simulink model "adaptive_beamforming"  (R2026a)
settings: Solver=VariableStepAuto  StopTime=60
libraries: dspstat3 x2, commchan3 x1, commfilt2 x1, commrandsrc3 x1, commdigbbndam3 x1
settings Model: PacingRate=4  Creator=Krrrrish  LastModifiedBy=swaja

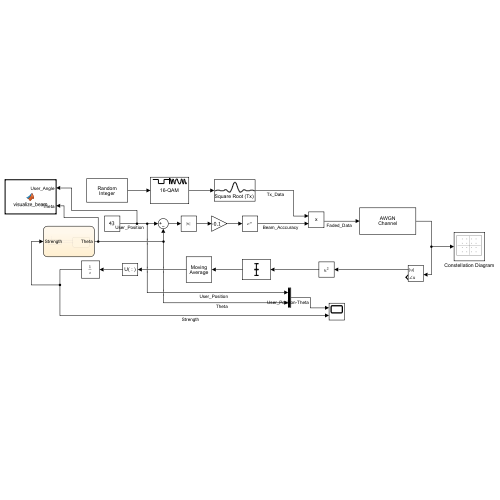
[thumbnail: Simulink's stored preview of the top-level diagram]
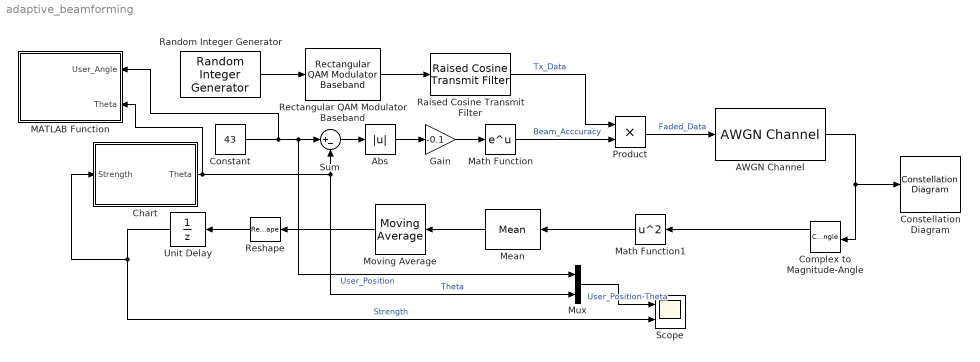
== system adaptive_beamforming ==
  AWGN Channel : commchan3/AWGN Channel  LegacyMode=off  NoiseMethod="Signal to noise ratio  (SNR)"  noiseMode="Signal to noise ratio  (SNR)"  EbNo=10  EsNo=10  SNR=10  BitsPerSymbol=1  SignalPower=1  SpecifySymbolPeriod=off  SamplesPerSymbol=1  SymbolPeriod=1  VarianceSource=Parameter  Variance=1  RandomStream=Global stream  Seed=67  SimulateUsing=Code generation
  Abs : Abs  SaturateOnIntegerOverflow=off
  Chart : Stateflow chart  TreatAsAtomicUnit=on
  Complex to Magnitude-Angle : ComplexToMagnitudeAngle
  Constant : Constant  Value=43
  Constellation Diagram : ConstellationDiagram  WindowPosition=[1071.000000,156.000000,600.000000,600.000000,]  ScopeFrameLocation=window  DefaultConfigurationName=comm.scopes.ConstellationDiagramBlockCfg
  Gain : Gain  Gain=-0.1
  MATLAB Function : MATLAB Function  TreatAsAtomicUnit=on
  Math Function : Math
  Math Function1 : Math  Operator=square
  Mean : dspstat3/Mean  run=off  InputProcessing=Columns as channels (frame based)  reset_popup=None  directionMode=Each column  dimension=1  roiEnable=off  roiType=Rectangles  roiPortion=Entire ROI  roiOutput=Individual statistics for each ROI  roiFlag=off  roundingMode=Floor  overflowMode=off  outputMin=[]  outputMax=[]
  Moving Average : dspstat3/Moving Average  Method=Sliding window  ForgettingFactorPort=off  SpecifyWindowLength=on  WindowLengthSource=Property  MaxWindowLength=20  WindowLength=4  OverlapLength=3  AllowArbitraryInputLength=off  ForgettingFactor=0.9  SimulateUsing=Interpreted execution
  Mux : Mux  Inputs=2
  Product : Product
  Raised Cosine Transmit Filter : commfilt2/Raised Cosine Transmit Filter  filtType=Square root  R=0.2  filtSpan=10  N=8  filterGain=1  InputProcessing=Columns as channels (frame based)  RateOptions=Enforce single-rate processing  framing=Mute  checkCoeff=off  variableName=rcTxFilt  checkGain=Normalized  sampMode=Mute  saveAsFlag=0  currentFiltSpan=10  D=(10)/2  launchFVT=on  roundingMode=Floor  overflowMode=off  coeffDataTypeStr=Inherit: Same word length as input  coeffMin=[]  coeffMax=[]  coeffLastDataTypeStr=Inherit: Same word length as input  outputDataTypeStr=Inherit: Same as accumulator  outputMin=[]  outputMax=[]  outputLastDataTypeStr=Inherit: Same as accumulator
  Random Integer Generator : commrandsrc3/Random Integer Generator  SetSize=8  SeedSource=Auto  Seed=0  SampleTime=1  SamplesPerFrame=1  OutputDataType=double  SimulateUsing=Interpreted execution
  Rectangular QAM Modulator Baseband : commdigbbndam3/Rectangular QAM Modulator Baseband  M=16  InType=Integer  Enc=Gray  Mapping=[0:15]  PowType=Min. distance between symbols  MinDist=2  AvgPow=1  PeakPow=1  Ph=0  outDtype=double  outWordLen=16  outUDDataType=sfix(16)  outFracLenMode=Best precision  outFracLen=15  outDataTypeStr=double  outLastDataTypeStr=double
  Reshape : Reshape
  Scope : Scope  NumInputPorts=2
      settings: ActiveDisplayYMinimum=-130.96926801320939  ActiveDisplayYMaximum=619.509013291859
  Sum : Sum  Inputs=|+-
  Unit Delay : UnitDelay  SampleTime=0.01
  wires:
  Random Integer Generator/1 -> Rectangular QAM Modulator Baseband/1
  Rectangular QAM Modulator Baseband/1 -> Raised Cosine Transmit Filter/1
  Raised Cosine Transmit Filter/1 -> Product/1  "Tx_Data"
  Chart/1(Theta) -> MATLAB Function/2(Theta), Mux/2, Sum/2  "Theta"
  Constant/1 -> MATLAB Function/1(User_Angle), Mux/1, Sum/1  "User_Position"
  Sum/1 -> Abs/1
  Abs/1 -> Gain/1
  Gain/1 -> Math Function/1
  Math Function/1 -> Product/2  "Beam_Acccuracy"
  Product/1 -> AWGN Channel/1  "Faded_Data"
  AWGN Channel/1 -> Constellation Diagram/1, Complex to Magnitude-Angle/1
  Complex to Magnitude-Angle/1 -> Math Function1/1
  Math Function1/1 -> Mean/1
  Mean/1 -> Moving Average/1
  Unit Delay/1 -> Scope/2, Chart/1(Strength)  "Strength"
  Reshape/1 -> Unit Delay/1
  Mux/1 -> Scope/1  "User_Position-Theta"
  Moving Average/1 -> Reshape/1

== matlab function adaptive_beamforming/MATLAB Function ==
  data: User_Angle input; Theta input
function visualize_beam(User_Angle, Theta)
    % This command tells Simulink to allow live MATLAB figure plotting
    coder.extrinsic('plot', 'scatter', 'axis', 'drawnow', 'hold', 'title');

    % 1. Create a 360-degree circle of angles
    phi = linspace(-180, 180, 360);

    % 2. Calculate the angle difference (with wrap-around math)
    diff = mod((phi - Theta) + 180, 360) - 180;

    % 3. Calculate the Beam Power (The Teardrop Shape)
    P = exp(-0.1 * (diff.^2));

    % 4. Convert Polar coordinates to Cartesian (X, Y for the graph)
    phi_rad = phi * (pi / 180);
    Beam_X = P .* cos(phi_rad);
    Beam_Y = P .* sin(phi_rad);

    % 5. Calculate the User's X, Y position
    % We set the radius to 1.1 so the red dot sits just slightly outside the beam
    User_rad = User_Angle * (pi / 180);
    User_X = 1.1 * cos(User_rad); 
    User_Y = 1.1 * sin(User_rad);

    % --- LIVE DRAWING COMMANDS ---
    plot(Beam_X, Beam_Y, 'b-', 'LineWidth', 2); 
    hold('on');
    scatter(User_X, User_Y, 150, 'r', 'filled');
    plot([0 User_X], [0 User_Y], 'r--');        
    
    axis([-1.2 1.2 -1.2 1.2]); 
    title('Live 5G Beam Tracking');
    hold('off');
    
    drawnow; % Forces the screen to refresh every single time step
end

== stateflow chart adaptive_beamforming/Chart ==
  state TRACK
    en:
    Search_Dir = 1;
    Lost_Count = 0;
    du:
    if (Strength < 0.2)
    Lost_Count = Lost_Count + 1;
    else
    Lost_Count = 0;
    end
    if (Strength < P_old)
    Search_Dir = -Search_Dir;
    end
    Theta = Theta + (Search_Dir * 0.2);
    P_old = Strength;
  state SEARCH
    en:
    Theta = -180;
    du:
    Theta = Theta + 1;
    if Theta > 180
    Theta = -180;
    end
  (default) -> SEARCH
  TRACK -> SEARCH : [Lost_Count > 10]
  SEARCH -> TRACK : [Strength > 0.8]
  data: Strength input; Theta output; P_old local size=1 =0; Search_Dir local; Lost_Count local size=1
